simulink model "nms_3Dmodel_forward"  (R2017b)
settings: Solver=VariableStepAuto  StartTime=0.0  StopTime=t_end  FixedStep=1e-4  MinStep=1e-9  RelTol=1e-2  AbsTol=1e-3  EnableMultiTasking=on
InitFcn:
  | runScripts;
values from neighbouring files (symbols this model uses):
  ankle_height = 0.08    [nms_MechInit.m]
  ankleIMP = param(91+length(paramIC_opt):93+length(paramIC_opt))    [runScripts.m]
  c = 0.05    [IID_nms_MechInit.m]    (also in nms_MechInit.m)
  c_jointstop = 0.3 / (pi/180)    (= 17.1887338539)    [IID_nms_MechInit.m]    (also in nms_MechInit.m)
  CPG_On = 0    [setCPGPar.m]    (also in setCPGPar_inv.m = 1)
  CtrlPar_FP = [alpha0 alpha_cd alpha_cv]    [setCtrlPar.m]
  CtrlPar_FP_R = [R_hipR0 R_hipR_cd R_hipR_cv]    [setCtrlPar.m]
  CtrlPar_LL = l_clr    [setCtrlPar.m]
  CtrlPar_Side = [beta_cd  beta_cv]    [setCtrlPar.m]
  CtrlPar_St = [StPreStim St_M1 St_M2 St_M3 St_M4 St_M5 St_M11]    [setCtrlPar.m]
  CtrlPar_St_R = [R_StPreStim R_St_M1 R_St_M3 R_St_M4]    [setCtrlPar.m]
  CtrlPar_Sw = [SwPreStim SwPhasePari SwPhaseParii SwCtrlPar_H SwCtrlPar_A      SwCtrlPar_Ki SwCtrlPar_Kii SwCtrlPar_Kiii SwCtrlPar_StP]    [setCtrlPar.m]
  CtrlPar_Sw_R = [R_SwPreStim R_Sw_M6]    [setCtrlPar.m]
  CtrlPar_theta0 = parBlCtrl(1)      *1*pi/180    [setCtrlPar.m]
  CtrlPar_Tr = [Tr_St_sup Tr_Sw]    [setCtrlPar.m]
  CtrlPar_Tr_R = [R_Tr_St_sup R_Tr_Sw]    [setCtrlPar.m]
  D12_F = 0.16    [IID_nms_MechInit.m]    (also in nms_MechInit.m)
  D12_S = L_S    (= 0.5)    [IID_nms_MechInit.m]    (also in nms_MechInit.m = 0.46)
  D12_T = L_T    (= 0.5)    [IID_nms_MechInit.m]    (also in nms_MechInit.m = 0.46)
  D12z_T = 0.1* scalorFactor    (= 0.1)    [nms_MechInit.m]
  D13_F = 0.20    (= 0.2)    [IID_nms_MechInit.m]    (also in nms_MechInit.m)
  D1G_F = 0.14    [IID_nms_MechInit.m]    (also in nms_MechInit.m)
  D1G_HAT = 0.35    [IID_nms_MechInit.m]    (also in nms_MechInit.m)
  D1G_S = 0.3    [IID_nms_MechInit.m]    (also in nms_MechInit.m = 0.28)
  D1G_T = 0.3    [IID_nms_MechInit.m]    (also in nms_MechInit.m = 0.28)
  D1Gy_F = ankle_height*D1G_F/D12_F    (= 0.07)    [nms_MechInit.m]
  d_fBall = 0.1    [nms_MechInit.m]
  d_fHeel = 0.05    [nms_MechInit.m]
  DeltaThRef = 5e-3    (= 0.005)    [IID_nms_MechInit.m]    (also in nms_MechInit.m)
  Dist_LM23_PH = 0    [setDistPar.m]
  Dist_LM34_PH = 0    [setDistPar.m]
  Dist_On = 1    [IID_setDistPar.m]    (also in setDistPar.m)
  Dist_PDur = 0.15    [IID_setDistPar.m]    (also in setDistPar.m)
  Dist_RM23_PH = 0    [setDistPar.m]
  Dist_RM34_PH = 0    [setDistPar.m]
  Dist_StartTime = 15    [IID_setDistPar.m]    (also in setDistPar.m)
  Dist_xyzHAT_front_PH = 0    [setDistPar.m]
  Dist_xyzHAT_sag_PH = 0    [IID_setDistPar.m]    (also in setDistPar.m)
  Dist_xyzLAnkle_PH = 0    [setDistPar.m]
  Dist_xyzRAnkle_PH = 0    [setDistPar.m]
  eref = 0.04    [IID_nms_MechInit.m]    (also in nms_MechInit.m)
  FmaxBFSH = 350    [nms_MechInit.m]
  FmaxGAS = 1500    [IID_nms_MechInit.m]    (also in nms_MechInit.m)
  FmaxGLU = 1500    [IID_nms_MechInit.m]    (also in nms_MechInit.m)
  FmaxHAB = 3000    [nms_MechInit.m]
  FmaxHAD = 4500    [nms_MechInit.m]
  FmaxHAM = 3000    [IID_nms_MechInit.m]    (also in nms_MechInit.m)
  FmaxHFL = 2000    [IID_nms_MechInit.m]    (also in nms_MechInit.m)
  FmaxRF = 1200    [nms_MechInit.m]
  FmaxSOL = 4000    [IID_nms_MechInit.m]    (also in nms_MechInit.m)
  FmaxTA = 800    [IID_nms_MechInit.m]    (also in nms_MechInit.m)
  FmaxVAS = 6000    [IID_nms_MechInit.m]    (also in nms_MechInit.m)
  In_F = 0.005    [IID_nms_MechInit.m]    (also in nms_MechInit.m)
  In_HAT = 3    [IID_nms_MechInit.m]    (also in nms_MechInit.m = 2.5)
  In_S = 0.05    [IID_nms_MechInit.m]    (also in nms_MechInit.m)
  In_T = 0.15    [IID_nms_MechInit.m]    (also in nms_MechInit.m)
  init_a_tgt = 70*pi/180    (= 1.2217304764)    [setInitPar.m]
  init_a_tgtR = 90*pi/180    (= 1.57079632679)    [setInitPar.m]
  Inx_F = 0.0007    [nms_MechInit.m]
  Inx_HAT = 1.0    (= 1)    [nms_MechInit.m]
  Inx_S = 0.003    [nms_MechInit.m]
  Inx_T = 0.03    [nms_MechInit.m]
  Iny_F = 0.005    [nms_MechInit.m]
  Iny_HAT = 4.0    (= 4)    [nms_MechInit.m]
  Iny_S = 0.05    [nms_MechInit.m]
  Iny_T = 0.15    [nms_MechInit.m]
  K = 5    [IID_nms_MechInit.m]    (also in nms_MechInit.m)
  k_gn = k_gn/2    (= 39240)    [nms_MechInit.m]
  k_gt = k_gt/2    (= 3924)    [nms_MechInit.m]
  k_pressure = m_HAT * 9.81 / DeltaThRef    (= 104967)    [IID_nms_MechInit.m]    (also in nms_MechInit.m)
  leg_l = [D12_T D12_S]    [nms_MechInit.m]
  LongDelay = 0.020    (= 0.02)    [IID_setCtrlPar.m]    (also in nms_MechInit.m = 0.01)
  LongLoopDelay = 0.030    (= 0.03)    [nms_MechInit.m]
  loptBFSH = 0.12    [nms_MechInit.m]
  loptGAS = 0.05    [IID_nms_MechInit.m]    (also in nms_MechInit.m)
  loptGLU = 0.11    [IID_nms_MechInit.m]    (also in nms_MechInit.m)
  loptHAB = 0.09    [nms_MechInit.m]
  loptHAD = 0.10    (= 0.1)    [nms_MechInit.m]
  loptHAM = 0.10    (= 0.1)    [IID_nms_MechInit.m]    (also in nms_MechInit.m)
  loptHFL = 0.11    [IID_nms_MechInit.m]    (also in nms_MechInit.m)
  loptRF = 0.08    [nms_MechInit.m]
  loptSOL = 0.04    [IID_nms_MechInit.m]    (also in nms_MechInit.m)
  loptTA = 0.06    [IID_nms_MechInit.m]    (also in nms_MechInit.m)
  loptVAS = 0.08    [IID_nms_MechInit.m]    (also in nms_MechInit.m)
  lslackBFSH = 0.10    (= 0.1)    [nms_MechInit.m]
  lslackGAS = 0.40    (= 0.4)    [IID_nms_MechInit.m]    (also in nms_MechInit.m)
  lslackGLU = 0.13    [IID_nms_MechInit.m]    (also in nms_MechInit.m)
  lslackHAB = 0.07    [nms_MechInit.m]
  lslackHAD = 0.18    [nms_MechInit.m]
  lslackHAM = 0.31    [IID_nms_MechInit.m]    (also in nms_MechInit.m)
  lslackHFL = 0.10    (= 0.1)    [IID_nms_MechInit.m]    (also in nms_MechInit.m)
  lslackRF = 0.35    [nms_MechInit.m]
  lslackSOL = 0.26    [IID_nms_MechInit.m]    (also in nms_MechInit.m)
  lslackTA = 0.24    [IID_nms_MechInit.m]    (also in nms_MechInit.m)
  lslackVAS = 0.23    [IID_nms_MechInit.m]    (also in nms_MechInit.m)
  m_F = 1.25    [IID_nms_MechInit.m]    (also in nms_MechInit.m)
  m_HAT = 53.5    [IID_nms_MechInit.m]    (also in nms_MechInit.m)
  m_S = 3.5    [IID_nms_MechInit.m]    (also in nms_MechInit.m)
  m_T = 8.5    [IID_nms_MechInit.m]    (also in nms_MechInit.m)
  m_Total = m_F*2+m_S*2+m_T*2+m_HAT    (= 80)    [IID_nms_MechInit.m]    (also in nms_MechInit.m)
  massBFSH = 2    [nms_MechInit.m]
  massGAS = 0.45    [IID_nms_MechInit.m]    (also in nms_MechInit.m)
  massGLU = 1.4    [IID_nms_MechInit.m]    (also in nms_MechInit.m)
  massHAB = 1.145    [nms_MechInit.m]
  massHAD = 1.91    [nms_MechInit.m]
  massHAM = 1.82    [IID_nms_MechInit.m]    (also in nms_MechInit.m)
  massHFL = 1.87    [IID_nms_MechInit.m]    (also in nms_MechInit.m)
  massRF = 1    [nms_MechInit.m]
  massSOL = 1.36    [IID_nms_MechInit.m]    (also in nms_MechInit.m)
  massTA = 0.29    [IID_nms_MechInit.m]    (also in nms_MechInit.m)
  massVAS = 2.91    [IID_nms_MechInit.m]    (also in nms_MechInit.m)
  MidDelay = 0.010    (= 0.01)    [IID_setCtrlPar.m]    (also in nms_MechInit.m = 0.005)
  mu_slide = 0.8    [IID_nms_MechInit.m]    (also in nms_MechInit.m)
  mu_stick = 0.9    [IID_nms_MechInit.m]    (also in nms_MechInit.m)
  N = 1.5    [IID_nms_MechInit.m]    (also in cmaes_parfor.m = size(x,1); nms_MechInit.m)
  phi12_LowLimit = 70*pi/180    (= 1.2217304764)    [IID_nms_MechInit.m]    (also in nms_MechInit.m)
  phi12_UpLimit = 130*pi/180    (= 2.26892802759)    [IID_nms_MechInit.m]    (also in nms_MechInit.m)
  phi23_UpLimit = 175*pi/180    (= 3.05432619099)    [IID_nms_MechInit.m]    (also in nms_MechInit.m)
  phi34_UpLimit = 230*pi/180    (= 4.01425727959)    [IID_nms_MechInit.m]    (also in nms_MechInit.m)
  phi34R_LowLimit = -15*pi/180    (= -0.261799387799)    [nms_MechInit.m]
  ... (+115 more)
undefined symbols (not defined in the file or in its folder): Control_type, Fs_prosthesis, magnitude, sgn
libraries: mblibv1 x104, simulink x54, simulink_extras x38, nmc x30, NMCCPG_Library x17, powerlib_meascontrol x5
(part 2 of 17)

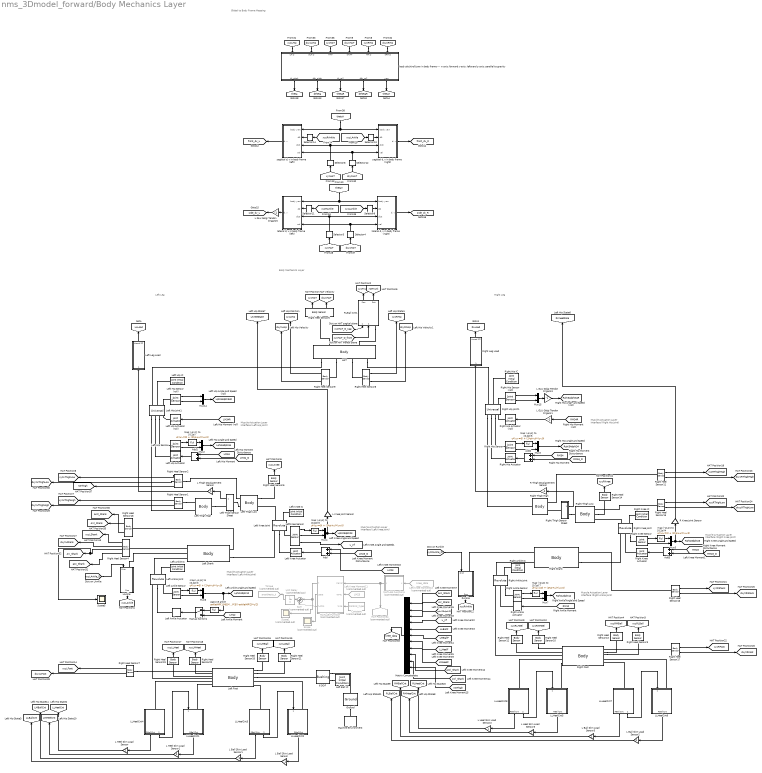
== system nms_3Dmodel_forward/Body Mechanics Layer ==
  note: Global to Body Frame Mapping
  note: Body Mechanics Layer
  note: Left Leg
  note: Right Leg
  note: Muscle Actuation
      | Layer Interface
      | (Left Hip Joint)
  note: Muscle Actuation
      | Layer Interface
      | (Left Knee Joint)
  note: Muscle Actuation
      | Layer Interface
      | (Left Ankle Joint)
  note: Muscle Actuation
      | Layer Interface
      | (Right Ankle Joint)
  note: Muscle Actuation
      | Layer Interface
      | (Right Knee Joint)
  note: Muscle Actuation
      | Layer Interface
      | (Right Hip Joint)
  6 DOF : mblibv1/Joints/Bushing  LConnTagsString=__newl0|SA1  RConnTagsString=__newr0  UpdateFromCAD=off  NumSAPorts=1  CutJoint=off  MarkAsCut=off  Primitives=prismatic_prismatic_prismatic  PrimitiveProps=P1$World$[1 0 0]$prismatic#P2$World$[0 1 0]$prismatic#P3$World$[0 0 1]$prismatic#R1$World$[1 0 0]$revolute#R2$World$[0 1 0]$revolute#R3$World$[0 0 1]$revolute  DialogClass=JointBlock  P1Axis=[1 0 0]  P2Axis=[0 1 0]  P3Axis=[0 0 1]  R1Axis=[1 0 0]  R2Axis=[0 1 0]  R3Axis=[0 0 1]
      settings: SourceProductName=Simscape Multibody  SourceProductBaseCode=MS
  Add{,1..3} (4 alike) : Sum
  Constant : Constant  Commented=on  Value=Control_type
  Ground : mblibv1/Bodies/Ground  UpdateFromCAD=off  LeftPortType=env  RightPortType=workingframe  PhysicalDomain=Mechanical  DialogClass=GroundBlock  CoordPosition=[0 0 0]  CoordPositionUnits=m  StateVectorMgrId=-1  MachineId=[0 0]  ShowEnvPort=on  ParameterChecksum=[4161457147, 3465215922, 4275957607, 1609472700]  TopologyChecksum=[2240496932, 2843436453, 1555863817, 2055023969]
      settings: SourceProductName=Simscape Multibody  SourceProductBaseCode=MS
  HAT : mblibv1/Bodies/Body  LConnTagsString=CG|CS6  RConnTagsString=CS1|CS2|CS3|CS4  UpdateFromCAD=off  DialogClass=MechanicalBodyBlock  Mass=m_HAT  MassUnits=kg  InertiaUnits=kg*m^2  Inertia=[Inx_HAT 0 0; 0 Iny_HAT 0; 0 0 In_HAT]  Shape=Cylinder  ShapeDims=[1 1]  ShapeUnits=m  ShapeUse=false  Density=1  DensityUnits=kg/m^3  DensityUse=false  GraphicsMode=MACHINE_DEFAULT  BodyColorSelMode=MACHINE_DEFAULT  BodyColor=[1 0 0]  AttachedToCS=CG  CG=Left$CG$[D1G_HAT 0 D12z_T]$CS1$CS1$m$[0 0 0]$Euler X-Y-Z$deg$WORLD$true$none  WorkingFrames=Left$CS5$[0.8 0 D12z_T]$CS1$CS1$m$[0 0 0]$Euler X-Y-Z$deg$WORLD$false$none#Right$CS1$[0 0 0]$ADJOINING$ADJOINING$m$[0 0 0]$Euler X-Y-Z$deg$WORLD$true$none#Right$CS2$[0 0 0]$CS1$CS1$m$[0 0 0]$Euler X-Y-Z$deg$WORLD$true$none#Right$CS3$[0 0 0]$CS4$CS4$m$[0 0 0]$Euler X-Y-Z$deg$WORLD$true$none#Right$CS4$[0 0 2*D12z_T]$CS1$CS1$m$[0 0 0]$Euler X-Y-Z$deg$WORLD$true$none#Left$CS6$[0 0 D12z_T]$CS1$CS1$m$[0 0 0]$Euler X-Y-Z$deg$WORLD$true$none  CGPos=[D1G_HAT 0 D12z_T]  CGRot=[0 0 0]  CS0Pos=[]  CS0Rot=[]  CS1Pos=[0 0 0]  CS1Rot=[0 0 0]  CS2Pos=[0 0 0]  CS2Rot=[0 0 0]  CS3Pos=[0 0 0]  CS3Rot=[0 0 0]  CS4Pos=[0 0 2*D12z_T]  CS4Rot=[0 0 0]  CS5Pos=[0.8 0 D12z_T]  CS5Rot=[0 0 0]  CS6Pos=[0 0 D12z_T]  CS6Rot=[0 0 0]  CS7Pos=[]  CS7Rot=[]  CS8Pos=[]  CS8Rot=[]  CS9Pos=[]  CS9Rot=[]  CS10Pos=[]  CS10Rot=[]  CS11Pos=[]  CS11Rot=[]  CS12Pos=[]  CS12Rot=[]  CS13Pos=[]  CS13Rot=[]  CS14Pos=[]  CS14Rot=[]  CS15Pos=[]  CS15Rot=[]  CS16Pos=[]  CS16Rot=[]  CS17Pos=[]  CS17Rot=[]  CS18Pos=[]  CS18Rot=[]  CS19Pos=[]  CS19Rot=[]  CS20Pos=[]  CS20Rot=[]
      settings: SourceProductName=Simscape Multibody  SourceProductBaseCode=MS
  HAT Position34 : Goto  Commented=on  GotoTag=knee_data_buffer  TagVisibility=global
  L Ball Skin Load Sensor{,1..3} (4 alike) : Gain
  L GLU Golgi Tendon Organs1 : Gain  Gain=-1
  L GLU Golgi Tendon Organs3 : Gain  Gain=-1
  L GLU Golgi Tendon Organs5 : Gain  Gain=-1
  L Heel Skin Load Sensor{,1..3} (4 alike) : Gain
  L Knee Joint Sensor : Gain
  L Thigh Displacement  Sensor : Gain
  LAnkle : Subsystem
  LLHeelCnt1 : Subsystem
  LLHeelCnt2 : Subsystem
  LLHeelCnt3 : Subsystem
  LLHeelCnt4 : Subsystem
  LLHeelCnt5 : Subsystem
  LLHeelCnt6 : Subsystem
  LLHeelCnt7 : Subsystem
  LLHeelCnt8 : Subsystem
  Left Ankle Joint : mblibv1/Joints/Revolute  LConnTagsString=__newl0|SA1|SA2  RConnTagsString=__newr0|SA1  UpdateFromCAD=off  NumSAPorts=3  CutJoint=off  MarkAsCut=off  Primitives=revolute  PrimitiveProps=R1$WORLD$[0 0 1]$revolute  DialogClass=JointBlock  R1Axis=[0 0 1]
      settings: SourceProductName=Simscape Multibody  SourceProductBaseCode=MS
  Left Hip Joint1 : mblibv1/Joints/Universal  LConnTagsString=__newl0|SA1|SA2|SA3  RConnTagsString=__newr0|SA1|SA2  UpdateFromCAD=off  NumSAPorts=5  CutJoint=off  MarkAsCut=off  Primitives=prismatic  PrimitiveProps=R1$World$[0 0 1]$revolute#R2$World$[0 1 0]$revolute  DialogClass=JointBlock  R1Axis=[0 0 1]  R2Axis=[0 1 0]
      settings: SourceProductName=Simscape Multibody  SourceProductBaseCode=MS
  Left Knee Joint : mblibv1/Joints/Revolute  LConnTagsString=__newl0|SA1|SA2  RConnTagsString=__newr0|SA1  UpdateFromCAD=off  NumSAPorts=3  CutJoint=off  MarkAsCut=off  Primitives=revolute  PrimitiveProps=R1$WORLD$[0 0 -1]$revolute  DialogClass=JointBlock  R1Axis=[0 0 -1]
      settings: SourceProductName=Simscape Multibody  SourceProductBaseCode=MS
  Left Ankle Actuator : mblibv1/Sensors &  Actuators/Joint Actuator  UpdateFromCAD=off  PhysicalDomain=Mechanical  PortType=blob  ActuationStyle=Force  AngleUnits=deg  ArcVelocityUnits=deg/s  ArcAccelerationUnits=deg/s^2  CoordPositionUnits=m  VelocityUnits=m/s  AccelerationUnits=m/s^2  ForceUnits=N  TorqueUnits=N-m  ActiveIO=on  Width=1  DialogClass=MechanicalActuatorBlock  Primitive=R1  ReferenceFrame=Absolute (INERTIAL)
      settings: SourceProductName=Simscape Multibody  SourceProductBaseCode=MS
  Left Ankle Sensor : mblibv1/Sensors &  Actuators/Joint Sensor  UpdateFromCAD=off  PhysicalDomain=Mechanical  PortType=blob  Muxed=off  Pose=off  Angle=on  AngleUnits=rad  ArcVelocity=on  ArcVelocityUnits=rad/s  ArcAcceleration=off  ArcAccelerationUnits=deg/s^2  CoordPosition=on  CoordPositionUnits=m  Velocity=off  VelocityUnits=m/s  Acceleration=off  AccelerationUnits=m/s^2  Quaternion=on  QuaternionDT=off  QuaternionDDT=off  QuaternionUnits=off  OutputVector=[ 1 1 ]  ActiveIO=on  Width=2  DialogClass=MechanicalSensorBlock  Primitive=R1  Force=off  ForceUnits=N  Torque=off  TorqueUnits=N-m  ReferenceFrame=Absolute (INERTIAL)  ReactionSensedSide=Base  ReactionReferenceFrame=Absolute (World)  ReactionForce=off  ReactionForceUnits=N  ReactionMoment=off  ReactionMomentUnits=N-m
      settings: SourceProductName=Simscape Multibody  SourceProductBaseCode=MS
  Left Ankle IC : mblibv1/Sensors &  Actuators/Joint Initial Condition  UpdateFromCAD=off  LeftPortType=blob  RightPortType=blob  PhysicalDomain=mechanical  DialogClass=InitialConditionBlock  InitialConditions=P1$false$0$m$rad$0$m/s$rad/s#P2$false$0$m$rad$0$m/s$rad/s#P3$false$0$m$rad$0$m/s$rad/s#R1$true$Lphi120$m$rad$0$m/s$rad/s#R2$false$0$m$rad$0$m/s$rad/s#R3$false$0$m$rad$0$m/s$rad/s#S$false$0$m$rad$0$m/s$rad/s  P1PIC=0  P1VIC=0  P2PIC=0  P2VIC=0  P3PIC=0  P3VIC=0  R1PIC=Lphi120  R1VIC=0  R2PIC=0  R2VIC=0  R3PIC=0  R3VIC=0  SPIC=0  SVIC=0
      settings: SourceProductName=Simscape Multibody  SourceProductBaseCode=MS
  Left Ball IC : mblibv1/Sensors &  Actuators/Joint Initial Condition  UpdateFromCAD=off  LeftPortType=blob  RightPortType=blob  PhysicalDomain=mechanical  DialogClass=InitialConditionBlock  InitialConditions=P1$true$x0$m$deg$vx0$m/s$deg/s#P2$true$z0$m$deg$0$m/s$deg/s#P3$true$-y0$m$deg$-vy0$m/s$deg/s#R1$true$roll0$m$rad$0$m/s$rad/s#R2$true$yaw0$m$rad$0$m/s$rad/s#R3$false$0$m$rad$0$m/s$rad/s#S$false$0$m$deg$0$m/s$deg/s  P1PIC=x0  P1VIC=vx0  P2PIC=z0  P2VIC=0  P3PIC=-y0  P3VIC=-vy0  R1PIC=roll0  R1VIC=0  R2PIC=yaw0  R2VIC=0  R3PIC=0  R3VIC=0  SPIC=0  SVIC=0
      settings: SourceProductName=Simscape Multibody  SourceProductBaseCode=MS
  Left Foot : mblibv1/Bodies/Body  LConnTagsString=CS3|CS4|CS1|CS5|CS6  RConnTagsString=CG|CS7|CS8|CS2|CS9|CS10  UpdateFromCAD=off  DialogClass=MechanicalBodyBlock  Mass=m_F  MassUnits=kg  InertiaUnits=kg*m^2  Inertia=[Inx_F 0 0; 0 Iny_F 0; 0 0 In_F]  Shape=Cylinder  ShapeDims=[1 1]  ShapeUnits=m  ShapeUse=false  Density=1  DensityUnits=kg/m^3  DensityUse=false  GraphicsMode=MACHINE_DEFAULT  BodyColorSelMode=MACHINE_DEFAULT  BodyColor=[1 0 0]  AttachedToCS=CG  CG=Right$CG$[-D1G_F D1Gy_F 0]$CS1$CS1$m$[0 0 0]$Euler X-Y-Z$deg$WORLD$true$none  WorkingFrames=Left$CS3$[0 0 d_fBall/2]$CS1$CS1$m$[0 0 0]$Euler X-Y-Z$deg$WORLD$true$none#Left$CS4$[0 0 -d_fBall/2]$CS1$CS1$m$[0 0 0]$Euler X-Y-Z$deg$WORLD$true$none#Right$CS7$[-D13_F 0 d_fHeel/2]$CS1$CS1$m$[0 0 0]$Euler X-Y-Z$deg$WORLD$true$none#Right$CS8$[-D13_F 0 -d_fHeel/2]$CS1$CS1$m$[0 0 0]$Euler X-Y-Z$deg$WORLD$true$none#Left$CS1$[0 0 0]$ADJOINING$ADJOINING$m$[0 0 0]$Euler X-Y-Z$deg$WORLD$true$none#Right$CS2$[-D12_F ankle_height 0]$CS1$CS1$m$[0 0 0]$Euler X-Y-Z$deg$WORLD$true$none#Left$CS5$[0 0 0]$CS4$CS4$m$[0 0 0]$Euler X-Y-Z$deg$WORLD$true$none#Left$CS6$[0 0 0]$CS3$CS3$m$[0 0 0]$Euler X-Y-Z$deg$WORLD$true$none#Right$CS9$[0 0 0]$CS8$CS8$m$[0 0 0]$Euler X-Y-Z$deg$WORLD$true$none#Right$CS10$[0 0 0]$CS7$CS7$m$[0 0 0]$Euler X-Y-Z$deg$WORLD$true$none  CGPos=[-D1G_F D1Gy_F 0]  CGRot=[0 0 0]  CS0Pos=[]  CS0Rot=[]  CS1Pos=[0 0 0]  CS1Rot=[0 0 0]  CS2Pos=[-D12_F ankle_height 0]  CS2Rot=[0 0 0]  CS3Pos=[0 0 d_fBall/2]  CS3Rot=[0 0 0]  CS4Pos=[0 0 -d_fBall/2]  CS4Rot=[0 0 0]  CS5Pos=[0 0 0]  CS5Rot=[0 0 0]  CS6Pos=[0 0 0]  CS6Rot=[0 0 0]  CS7Pos=[-D13_F 0 d_fHeel/2]  CS7Rot=[0 0 0]  CS8Pos=[-D13_F 0 -d_fHeel/2]  CS8Rot=[0 0 0]  CS9Pos=[0 0 0]  CS9Rot=[0 0 0]  CS10Pos=[0 0 0]  CS10Rot=[0 0 0]  CS11Pos=[]  CS11Rot=[]  CS12Pos=[]  CS12Rot=[]  CS13Pos=[]  CS13Rot=[]  CS14Pos=[]  CS14Rot=[]  CS15Pos=[]  CS15Rot=[]  CS16Pos=[]  CS16Rot=[]  CS17Pos=[]  CS17Rot=[]  CS18Pos=[]  CS18Rot=[]  CS19Pos=[]  CS19Rot=[]  CS20Pos=[]  CS20Rot=[]
      settings: SourceProductName=Simscape Multibody  SourceProductBaseCode=MS
  Left Hip Actuator : mblibv1/Sensors &  Actuators/Joint Actuator  UpdateFromCAD=off  PhysicalDomain=Mechanical  PortType=blob  ActuationStyle=Force  AngleUnits=deg  ArcVelocityUnits=deg/s  ArcAccelerationUnits=deg/s^2  CoordPositionUnits=m  VelocityUnits=m/s  AccelerationUnits=m/s^2  ForceUnits=N  TorqueUnits=N-m  ActiveIO=on  Width=1  DialogClass=MechanicalActuatorBlock  Primitive=R1  ReferenceFrame=Absolute (INERTIAL)
      settings: SourceProductName=Simscape Multibody  SourceProductBaseCode=MS
  Left Hip Actuator (roll) : mblibv1/Sensors &  Actuators/Joint Actuator  UpdateFromCAD=off  PhysicalDomain=Mechanical  PortType=blob  ActuationStyle=Force  AngleUnits=rad  ArcVelocityUnits=rad/s  ArcAccelerationUnits=rad/s^2  CoordPositionUnits=m  VelocityUnits=m/s  AccelerationUnits=m/s^2  ForceUnits=N  TorqueUnits=N*m  ActiveIO=on  Width=1  DialogClass=MechanicalActuatorBlock  Primitive=R2  ReferenceFrame=Absolute (INERTIAL)
      settings: SourceProductName=Simscape Multibody  SourceProductBaseCode=MS
  Left Hip Sensor : mblibv1/Sensors &  Actuators/Joint Sensor  UpdateFromCAD=off  PhysicalDomain=Mechanical  PortType=blob  Muxed=off  Pose=off  Angle=on  AngleUnits=rad  ArcVelocity=on  ArcVelocityUnits=rad/s  ArcAcceleration=off  ArcAccelerationUnits=deg/s^2  CoordPosition=on  CoordPositionUnits=m  Velocity=on  VelocityUnits=m/s  Acceleration=off  AccelerationUnits=m/s^2  Quaternion=on  QuaternionDT=off  QuaternionDDT=off  QuaternionUnits=off  OutputVector=[ 1 1 ]  ActiveIO=on  Width=2  DialogClass=MechanicalSensorBlock  Primitive=R1  Force=off  ForceUnits=N  Torque=off  TorqueUnits=N-m  ReferenceFrame=Absolute (INERTIAL)  ReactionSensedSide=Base  ReactionReferenceFrame=Absolute (World)  ReactionForce=off  ReactionForceUnits=N  ReactionMoment=off  ReactionMomentUnits=N-m
      settings: SourceProductName=Simscape Multibody  SourceProductBaseCode=MS
  Left Hip Sensor (roll) : mblibv1/Sensors &  Actuators/Joint Sensor  UpdateFromCAD=off  PhysicalDomain=Mechanical  PortType=blob  Muxed=off  Pose=off  Angle=on  AngleUnits=rad  ArcVelocity=on  ArcVelocityUnits=rad/s  ArcAcceleration=off  ArcAccelerationUnits=deg/s^2  CoordPosition=on  CoordPositionUnits=m  Velocity=on  VelocityUnits=m/s  Acceleration=off  AccelerationUnits=m/s^2  Quaternion=on  QuaternionDT=off  QuaternionDDT=off  QuaternionUnits=off  OutputVector=[ 1 1 ]  ActiveIO=on  Width=2  DialogClass=MechanicalSensorBlock  Primitive=R2  Force=off  ForceUnits=N  Torque=off  TorqueUnits=N*m  ReferenceFrame=Absolute (INERTIAL)  ReactionSensedSide=Base  ReactionReferenceFrame=Absolute (World)  ReactionForce=off  ReactionForceUnits=N  ReactionMoment=off  ReactionMomentUnits=N*m
      settings: SourceProductName=Simscape Multibody  SourceProductBaseCode=MS
  Left Hip IC : mblibv1/Sensors &  Actuators/Joint Initial Condition  UpdateFromCAD=off  LeftPortType=blob  RightPortType=blob  PhysicalDomain=mechanical  DialogClass=InitialConditionBlock  InitialConditions=P1$false$0$m$rad$0$m/s$rad/s#P2$false$0$m$rad$0$m/s$rad/s#P3$false$0$m$rad$0$m/s$rad/s#R1$true$Lphi340$m$rad$0$m/s$rad/s#R2$true$Lphi340R$m$rad$0$m/s$rad/s#R3$false$0$m$rad$0$m/s$rad/s#S$false$0$m$rad$0$m/s$rad/s  P1PIC=0  P1VIC=0  P2PIC=0  P2VIC=0  P3PIC=0  P3VIC=0  R1PIC=Lphi340  R1VIC=0  R2PIC=Lphi340R  R2VIC=0  R3PIC=0  R3VIC=0  SPIC=0  SVIC=0
      settings: SourceProductName=Simscape Multibody  SourceProductBaseCode=MS
  Left Knee Actuator : mblibv1/Sensors &  Actuators/Joint Actuator  UpdateFromCAD=off  PhysicalDomain=Mechanical  PortType=blob  ActuationStyle=Force  AngleUnits=deg  ArcVelocityUnits=deg/s  ArcAccelerationUnits=deg/s^2  CoordPositionUnits=m  VelocityUnits=m/s  AccelerationUnits=m/s^2  ForceUnits=N  TorqueUnits=N-m  ActiveIO=on  Width=1  DialogClass=MechanicalActuatorBlock  Primitive=R1  ReferenceFrame=Absolute (INERTIAL)
      settings: SourceProductName=Simscape Multibody  SourceProductBaseCode=MS
  Left Knee Moment11 : From  Commented=on  GotoTag=LM23  TagVisibility=global
      settings: CloseFcn=tagdialog Close
  Left Knee Moment13 : From  Commented=on  GotoTag=knee_data  TagVisibility=global
      settings: CloseFcn=tagdialog Close
  Left Knee IC : mblibv1/Sensors &  Actuators/Joint Initial Condition  UpdateFromCAD=off  LeftPortType=blob  RightPortType=blob  PhysicalDomain=mechanical  DialogClass=InitialConditionBlock  InitialConditions=P1$false$0$m$rad$0$m/s$rad/s#P2$false$0$m$rad$0$m/s$rad/s#P3$false$0$m$rad$0$m/s$rad/s#R1$true$Lphi230$m$rad$0$m/s$deg/s#R2$false$0$m$rad$0$m/s$rad/s#R3$false$0$m$rad$0$m/s$rad/s#S$false$0$m$rad$0$m/s$rad/s  P1PIC=0  P1VIC=0  P2PIC=0  P2VIC=0  P3PIC=0  P3VIC=0  R1PIC=Lphi230  R1VIC=0  R2PIC=0  R2VIC=0  R3PIC=0  R3VIC=0  SPIC=0  SVIC=0
      settings: SourceProductName=Simscape Multibody  SourceProductBaseCode=MS
  Left Leg Load : Subsystem
  Left Shank : mblibv1/Bodies/Body  LConnTagsString=CG|CS3|CS1  RConnTagsString=CS4|CS2  UpdateFromCAD=off  DialogClass=MechanicalBodyBlock  Mass=m_S  MassUnits=kg  InertiaUnits=kg*m^2  Inertia=[Inx_S 0 0; 0 Iny_S 0; 0 0 In_S]  Shape=Cylinder  ShapeDims=[1 1]  ShapeUnits=m  ShapeUse=false  Density=1  DensityUnits=kg/m^3  DensityUse=false  GraphicsMode=MACHINE_DEFAULT  BodyColorSelMode=MACHINE_DEFAULT  BodyColor=[1 0 0]  AttachedToCS=CG  CG=Left$CG$[D1G_S 0 0]$CS1$CS1$m$[0 0 0]$Euler X-Y-Z$deg$WORLD$true$none  WorkingFrames=Right$CS4$[D1G_S 0 0]$CS1$CS1$m$[0 0 0]$Euler X-Y-Z$deg$WORLD$true$none#Left$CS3$[0 0 0]$CS1$CS1$m$[0 0 0]$Euler X-Y-Z$deg$WORLD$true$none#Left$CS1$[0 0 0]$ADJOINING$ADJOINING$m$[0 0 0]$Euler X-Y-Z$deg$WORLD$true$none#Right$CS2$[D12_S 0 0]$CS1$CS1$m$[0 0 0]$Euler X-Y-Z$deg$WORLD$true$none  CGPos=[D1G_S 0 0]  CGRot=[0 0 0]  CS0Pos=[]  CS0Rot=[]  CS1Pos=[0 0 0]  CS1Rot=[0 0 0]  CS2Pos=[D12_S 0 0]  CS2Rot=[0 0 0]  CS3Pos=[0 0 0]  CS3Rot=[0 0 0]  CS4Pos=[D1G_S 0 0]  CS4Rot=[0 0 0]  CS5Pos=[]  CS5Rot=[]  CS6Pos=[]  CS6Rot=[]  CS7Pos=[]  CS7Rot=[]  CS8Pos=[]  CS8Rot=[]  CS9Pos=[]  CS9Rot=[]  CS10Pos=[]  CS10Rot=[]  CS11Pos=[]  CS11Rot=[]  CS12Pos=[]  CS12Rot=[]  CS13Pos=[]  CS13Rot=[]  CS14Pos=[]  CS14Rot=[]  CS15Pos=[]  CS15Rot=[]  CS16Pos=[]  CS16Rot=[]  CS17Pos=[]  CS17Rot=[]  CS18Pos=[]  CS18Rot=[]  CS19Pos=[]  CS19Rot=[]  CS20Pos=[]  CS20Rot=[]
      settings: SourceProductName=Simscape Multibody  SourceProductBaseCode=MS
  Left Thigh Sensor Sheet : Subsystem
  Left Thigh High : mblibv1/Bodies/Body  LConnTagsString=CG|CS2  RConnTagsString=CS1  UpdateFromCAD=off  DialogClass=MechanicalBodyBlock  Mass=m_T*(1-ThPos)  MassUnits=kg  InertiaUnits=kg*m^2  Inertia=[Inx_T*(1-ThPos) 0 0; 0 Iny_T*(1-ThPos)^3 0; 0 0 In_T*(1-ThPos)^3]  Shape=Cylinder  ShapeDims=[1 1]  ShapeUnits=m  ShapeUse=false  Density=1  DensityUnits=kg/m^3  DensityUse=false  GraphicsMode=MACHINE_DEFAULT  BodyColorSelMode=MACHINE_DEFAULT  BodyColor=[1 0 0]  AttachedToCS=CG  CG=Left$CG$[-D1G_T*(1-ThPos) 0 0]$CS1$CS1$m$[0 0 0]$Euler X-Y-Z$deg$WORLD$true$none  WorkingFrames=Right$CS1$[0 0 0]$ADJOINING$ADJOINING$m$[0 0 0]$Euler X-Y-Z$deg$WORLD$true$none#Left$CS2$[-D12_T*(1-ThPos) 0 0]$CS1$CS1$m$[0 0 0]$Euler X-Y-Z$deg$WORLD$true$none  CGPos=[-D1G_T*(1-ThPos) 0 0]  CGRot=[0 0 0]  CS0Pos=[]  CS0Rot=[]  CS1Pos=[0 0 0]  CS1Rot=[0 0 0]  CS2Pos=[-D12_T*(1-ThPos) 0 0]  CS2Rot=[0 0 0]  CS3Pos=[]  CS3Rot=[]  CS4Pos=[]  CS4Rot=[]  CS5Pos=[]  CS5Rot=[]  CS6Pos=[]  CS6Rot=[]  CS7Pos=[]  CS7Rot=[]  CS8Pos=[]  CS8Rot=[]  CS9Pos=[]  CS9Rot=[]  CS10Pos=[]  CS10Rot=[]  CS11Pos=[]  CS11Rot=[]  CS12Pos=[]  CS12Rot=[]  CS13Pos=[]  CS13Rot=[]  CS14Pos=[]  CS14Rot=[]  CS15Pos=[]  CS15Rot=[]  CS16Pos=[]  CS16Rot=[]  CS17Pos=[]  CS17Rot=[]  CS18Pos=[]  CS18Rot=[]  CS19Pos=[]  CS19Rot=[]  CS20Pos=[]  CS20Rot=[]
      settings: SourceProductName=Simscape Multibody  SourceProductBaseCode=MS
  Left Thigh Low : mblibv1/Bodies/Body  LConnTagsString=CG|CS2  RConnTagsString=CS3|CS1  UpdateFromCAD=off  DialogClass=MechanicalBodyBlock  Mass=m_T*ThPos  MassUnits=kg  InertiaUnits=kg*m^2  Inertia=[Inx_T*ThPos 0 0; 0 Iny_T*(ThPos)^3 0; 0 0 In_T*(ThPos)^3]  Shape=Cylinder  ShapeDims=[1 1]  ShapeUnits=m  ShapeUse=false  Density=1  DensityUnits=kg/m^3  DensityUse=false  GraphicsMode=MACHINE_DEFAULT  BodyColorSelMode=MACHINE_DEFAULT  BodyColor=[1 0 0]  AttachedToCS=CG  CG=Left$CG$[-D1G_T*ThPos 0 0]$CS1$CS1$m$[0 0 0]$Euler X-Y-Z$deg$WORLD$true$none  WorkingFrames=Right$CS3$[0 0 0]$CS1$CS1$m$[0 0 0]$Euler X-Y-Z$deg$WORLD$true$none#Right$CS1$[0 0 0]$ADJOINING$ADJOINING$m$[0 0 0]$Euler X-Y-Z$deg$WORLD$true$none#Left$CS2$[-D12_T*ThPos 0 0]$CS1$CS1$m$[0 0 0]$Euler X-Y-Z$deg$WORLD$true$none  CGPos=[-D1G_T*ThPos 0 0]  CGRot=[0 0 0]  CS0Pos=[]  CS0Rot=[]  CS1Pos=[0 0 0]  CS1Rot=[0 0 0]  CS2Pos=[-D12_T*ThPos 0 0]  CS2Rot=[0 0 0]  CS3Pos=[0 0 0]  CS3Rot=[0 0 0]  CS4Pos=[]  CS4Rot=[]  CS5Pos=[]  CS5Rot=[]  CS6Pos=[]  CS6Rot=[]  CS7Pos=[]  CS7Rot=[]  CS8Pos=[]  CS8Rot=[]  CS9Pos=[]  CS9Rot=[]  CS10Pos=[]  CS10Rot=[]  CS11Pos=[]  CS11Rot=[]  CS12Pos=[]  CS12Rot=[]  CS13Pos=[]  CS13Rot=[]  CS14Pos=[]  CS14Rot=[]  CS15Pos=[]  CS15Rot=[]  CS16Pos=[]  CS16Rot=[]  CS17Pos=[]  CS17Rot=[]  CS18Pos=[]  CS18Rot=[]  CS19Pos=[]  CS19Rot=[]  CS20Pos=[]  CS20Rot=[]
      settings: SourceProductName=Simscape Multibody  SourceProductBaseCode=MS
  LeftKnee Sensor : mblibv1/Sensors &  Actuators/Joint Sensor  UpdateFromCAD=off  PhysicalDomain=Mechanical  PortType=blob  Muxed=off  Pose=off  Angle=on  AngleUnits=rad  ArcVelocity=on  ArcVelocityUnits=rad/s  ArcAcceleration=off  ArcAccelerationUnits=deg/s^2  CoordPosition=on  CoordPositionUnits=m  Velocity=off  VelocityUnits=m/s  Acceleration=off  AccelerationUnits=m/s^2  Quaternion=on  QuaternionDT=off  QuaternionDDT=off  QuaternionUnits=off  OutputVector=[ 1 1 ]  ActiveIO=on  Width=5  DialogClass=MechanicalSensorBlock  Primitive=R1  Force=off  ForceUnits=N  Torque=off  TorqueUnits=N*m  ReferenceFrame=Absolute (INERTIAL)  ReactionSensedSide=Base  ReactionReferenceFrame=Absolute (World)  ReactionForce=on  ReactionForceUnits=N  ReactionMoment=off  ReactionMomentUnits=N*m
      settings: SourceProductName=Simscape Multibody  SourceProductBaseCode=MS
  MATLAB Function : MATLAB Function  Commented=on  TreatAsAtomicUnit=on
  MATLAB Function1 : MATLAB Function  Commented=on  TreatAsAtomicUnit=on
  Machine Environment : mblibv1/Bodies/Machine Environment  Tag=Factory ground  PortType=env  PhysicalDomain=Mechanical  DialogTemplateClass=MECH.MachineEnvironment  SyncWhenCopied=off  Gravity=[0 -9.81 0]  GravityUnits=m/s^2  GravityAsSignal=off  Dimensionality=3D Only  AnalysisType=Forward dynamics  LinearAssemblyTolerance=1e-3  LinearAssemblyToleranceUnits=m  AngularAssemblyTolerance=1e-3  AngularAssemblyToleranceUnits=rad  ConstraintSolverType=Tolerancing  ConstraintRelTolerance=1e-3  ConstraintAbsTolerance=1e-3  UseRobustSingularityHandling=off  RedundancyAnalysisToleranceType=Automatically select tolerance  RedundancyAnalysisTolerance=1e-14  StatePerturbationType=Fixed  PerturbationSize=1e-3  VisualizeMachine=on  BodyVisualizationType=Use model default body geometries  BodyColorSelMode=Use model default  DefaultBodyColor=[1 0.65 0]
      settings: SourceProductName=Simscape Multibody  SourceProductBaseCode=MS
  Manual Switch1 : ManualSwitch
  Matrix Concatenate : Concatenate  NumInputs=11  ConcatenateDimension=2
  Mux{2..7,14..15} (8 alike) : Mux  Inputs=2
  R Knee Joint Sensor : Gain
  R Thigh Displacement  Sensor : Gain  Gain=-1
  RAnkle : Subsystem
  RLBall Cnt1 : Subsystem
  Right Ankle Joint : mblibv1/Joints/Revolute  LConnTagsString=__newl0|SA1|SA2  RConnTagsString=__newr0|SA1  UpdateFromCAD=off  NumSAPorts=3  CutJoint=off  MarkAsCut=off  Primitives=revolute  PrimitiveProps=R1$WORLD$[0 0 1]$revolute  DialogClass=JointBlock  R1Axis=[0 0 1]
      settings: SourceProductName=Simscape Multibody  SourceProductBaseCode=MS
  Right Hip Joint1 : mblibv1/Joints/Universal  LConnTagsString=__newl0|SA1|SA2|SA3  RConnTagsString=__newr0|SA1|SA2  UpdateFromCAD=off  NumSAPorts=5  CutJoint=off  MarkAsCut=off  Primitives=prismatic  PrimitiveProps=R1$World$[0 0 1]$revolute#R2$World$[0 1 0]$revolute  DialogClass=JointBlock  R1Axis=[0 0 1]  R2Axis=[0 1 0]
      settings: SourceProductName=Simscape Multibody  SourceProductBaseCode=MS
  Right Knee Joint : mblibv1/Joints/Revolute  LConnTagsString=__newl0|SA1|SA2  RConnTagsString=__newr0|SA1  UpdateFromCAD=off  NumSAPorts=3  CutJoint=off  MarkAsCut=off  Primitives=revolute  PrimitiveProps=R1$WORLD$[0 0 -1]$revolute  DialogClass=JointBlock  R1Axis=[0 0 -1]
      settings: SourceProductName=Simscape Multibody  SourceProductBaseCode=MS
  Right Ankle Actuator : mblibv1/Sensors &  Actuators/Joint Actuator  UpdateFromCAD=off  PhysicalDomain=Mechanical  PortType=blob  ActuationStyle=Force  AngleUnits=deg  ArcVelocityUnits=deg/s  ArcAccelerationUnits=deg/s^2  CoordPositionUnits=m  VelocityUnits=m/s  AccelerationUnits=m/s^2  ForceUnits=N  TorqueUnits=N-m  ActiveIO=on  Width=1  DialogClass=MechanicalActuatorBlock  Primitive=R1  ReferenceFrame=Absolute (INERTIAL)
      settings: SourceProductName=Simscape Multibody  SourceProductBaseCode=MS
  Right Ankle Sensor : mblibv1/Sensors &  Actuators/Joint Sensor  UpdateFromCAD=off  PhysicalDomain=Mechanical  PortType=blob  Muxed=off  Pose=off  Angle=on  AngleUnits=rad  ArcVelocity=on  ArcVelocityUnits=rad/s  ArcAcceleration=off  ArcAccelerationUnits=deg/s^2  CoordPosition=on  CoordPositionUnits=m  Velocity=off  VelocityUnits=m/s  Acceleration=off  AccelerationUnits=m/s^2  Quaternion=on  QuaternionDT=off  QuaternionDDT=off  QuaternionUnits=off  OutputVector=[ 1 1 ]  ActiveIO=on  Width=2  DialogClass=MechanicalSensorBlock  Primitive=R1  Force=off  ForceUnits=N  Torque=off  TorqueUnits=N-m  ReferenceFrame=Absolute (INERTIAL)  ReactionSensedSide=Base  ReactionReferenceFrame=Absolute (World)  ReactionForce=off  ReactionForceUnits=N  ReactionMoment=off  ReactionMomentUnits=N-m
      settings: SourceProductName=Simscape Multibody  SourceProductBaseCode=MS
  Right Ankle IC : mblibv1/Sensors &  Actuators/Joint Initial Condition  UpdateFromCAD=off  LeftPortType=blob  RightPortType=blob  PhysicalDomain=mechanical  DialogClass=InitialConditionBlock  InitialConditions=P1$false$0$m$rad$0$m/s$rad/s#P2$false$0$m$rad$0$m/s$rad/s#P3$false$0$m$rad$0$m/s$rad/s#R1$true$Rphi120$m$rad$0$m/s$rad/s#R2$false$0$m$rad$0$m/s$rad/s#R3$false$0$m$rad$0$m/s$rad/s#S$false$0$m$rad$0$m/s$rad/s  P1PIC=0  P1VIC=0  P2PIC=0  P2VIC=0  P3PIC=0  P3VIC=0  R1PIC=Rphi120  R1VIC=0  R2PIC=0  R2VIC=0  R3PIC=0  R3VIC=0  SPIC=0  SVIC=0
      settings: SourceProductName=Simscape Multibody  SourceProductBaseCode=MS
  Right Foot : mblibv1/Bodies/Body  LConnTagsString=CG|CS3|CS4|CS2|CS5|CS6  RConnTagsString=CS7|CS8|CS1|CS9|CS10  UpdateFromCAD=off  DialogClass=MechanicalBodyBlock  Mass=m_F  MassUnits=kg  InertiaUnits=kg*m^2  Inertia=[Inx_F 0 0; 0 Iny_F 0; 0 0 In_F]  Shape=Cylinder  ShapeDims=[1 1]  ShapeUnits=m  ShapeUse=false  Density=1  DensityUnits=kg/m^3  DensityUse=false  GraphicsMode=MACHINE_DEFAULT  BodyColorSelMode=MACHINE_DEFAULT  BodyColor=[1 0 0]  AttachedToCS=CG  CG=Left$CG$[-D1G_F D1Gy_F 0]$CS2$CS2$m$[0 0 0]$Euler X-Y-Z$deg$WORLD$true$none  WorkingFrames=Left$CS3$[0 0 -d_fBall/2]$CS2$CS2$m$[0 0 0]$Euler X-Y-Z$deg$WORLD$true$none#Left$CS4$[0 0 d_fBall/2]$CS2$CS2$m$[0 0 0]$Euler X-Y-Z$deg$WORLD$true$none#Right$CS7$[-D13_F 0 -d_fHeel/2]$CS2$CS2$m$[0 0 0]$Euler X-Y-Z$deg$WORLD$true$none#Right$CS8$[-D13_F 0 d_fHeel/2]$CS2$CS2$m$[0 0 0]$Euler X-Y-Z$deg$WORLD$true$none#Right$CS1$[0 0 0]$ADJOINING$ADJOINING$m$[0 0 0]$Euler X-Y-Z$deg$WORLD$true$none#Left$CS2$[D12_F -ankle_height 0]$CS1$CS1$m$[0 0 0]$Euler X-Y-Z$deg$WORLD$true$none#Left$CS5$[0 0 0]$CS4$CS4$m$[0 0 0]$Euler X-Y-Z$deg$WORLD$true$none#Left$CS6$[0 0 0]$CS3$CS3$m$[0 0 0]$Euler X-Y-Z$deg$WORLD$true$none#Right$CS9$[0 0 0]$CS8$CS8$m$[0 0 0]$Euler X-Y-Z$deg$WORLD$true$none#Right$CS10$[0 0 0]$CS7$CS7$m$[0 0 0]$Euler X-Y-Z$deg$WORLD$true$none  CGPos=[-D1G_F D1Gy_F 0]  CGRot=[0 0 0]  CS0Pos=[]  CS0Rot=[]  CS1Pos=[0 0 0]  CS1Rot=[0 0 0]  CS2Pos=[D12_F -ankle_height 0]  CS2Rot=[0 0 0]  CS3Pos=[0 0 -d_fBall/2]  CS3Rot=[0 0 0]  CS4Pos=[0 0 d_fBall/2]  CS4Rot=[0 0 0]  CS5Pos=[0 0 0]  CS5Rot=[0 0 0]  CS6Pos=[0 0 0]  CS6Rot=[0 0 0]  CS7Pos=[-D13_F 0 -d_fHeel/2]  CS7Rot=[0 0 0]  CS8Pos=[-D13_F 0 d_fHeel/2]  CS8Rot=[0 0 0]  CS9Pos=[0 0 0]  CS9Rot=[0 0 0]  CS10Pos=[0 0 0]  CS10Rot=[0 0 0]  CS11Pos=[]  CS11Rot=[]  CS12Pos=[]  CS12Rot=[]  CS13Pos=[]  CS13Rot=[]  CS14Pos=[]  CS14Rot=[]  CS15Pos=[]  CS15Rot=[]  CS16Pos=[]  CS16Rot=[]  CS17Pos=[]  CS17Rot=[]  CS18Pos=[]  CS18Rot=[]  CS19Pos=[]  CS19Rot=[]  CS20Pos=[]  CS20Rot=[]
      settings: SourceProductName=Simscape Multibody  SourceProductBaseCode=MS
  Right Heel Sensor{1,5,7..9,11,15..17} (9 alike) : mblibv1/Sensors &  Actuators/Body Sensor  UpdateFromCAD=off  PhysicalDomain=Mechanical  PortType=blob  Muxed=off  Pose=off  Angle=on  AngleUnits=deg  ArcVelocity=off  ArcVelocityUnits=deg/s  ArcAcceleration=off  ArcAccelerationUnits=deg/s^2  CoordPosition=on  CoordPositionUnits=m  Velocity=on  VelocityUnits=m/s  Acceleration=off  AccelerationUnits=m/s^2  Quaternion=on  QuaternionDT=off  QuaternionDDT=off  QuaternionUnits=off  OutputVector=[ 3 3 ]  ActiveIO=on  Width=6  DialogClass=MechanicalSensorBlock  ReferenceFrame=Absolute (World)
      settings: SourceProductName=Simscape Multibody  SourceProductBaseCode=MS
  Right Heel Sensor{3,6,10,12..14,20..23} (10 alike) : mblibv1/Sensors &  Actuators/Body Sensor  UpdateFromCAD=off  PhysicalDomain=Mechanical  PortType=blob  Muxed=off  Pose=off  Angle=on  AngleUnits=deg  ArcVelocity=off  ArcVelocityUnits=deg/s  ArcAcceleration=off  ArcAccelerationUnits=deg/s^2  CoordPosition=on  CoordPositionUnits=m  Velocity=off  VelocityUnits=m/s  Acceleration=off  AccelerationUnits=m/s^2  Quaternion=on  QuaternionDT=off  QuaternionDDT=off  QuaternionUnits=off  OutputVector=[ 3 3 ]  ActiveIO=on  Width=3  DialogClass=MechanicalSensorBlock  ReferenceFrame=Absolute (World)
      settings: SourceProductName=Simscape Multibody  SourceProductBaseCode=MS
  Right Heel Sensor18 : mblibv1/Sensors &  Actuators/Body Sensor  UpdateFromCAD=off  PhysicalDomain=Mechanical  PortType=blob  Muxed=off  Pose=off  Angle=on  AngleUnits=deg  ArcVelocity=on  ArcVelocityUnits=deg/s  ArcAcceleration=off  ArcAccelerationUnits=deg/s^2  CoordPosition=off  CoordPositionUnits=m  Velocity=off  VelocityUnits=m/s  Acceleration=on  AccelerationUnits=m/s^2  Quaternion=on  QuaternionDT=off  QuaternionDDT=off  QuaternionUnits=off  OutputVector=[ 3 3 ]  ActiveIO=on  Width=6  DialogClass=MechanicalSensorBlock  ReferenceFrame=Local (Body CS)
      settings: SourceProductName=Simscape Multibody  SourceProductBaseCode=MS
  Right Heel Sensor2 : mblibv1/Sensors &  Actuators/Body Sensor  UpdateFromCAD=off  PhysicalDomain=Mechanical  PortType=blob  Muxed=off  Pose=on  Angle=on  AngleUnits=deg  ArcVelocity=off  ArcVelocityUnits=deg/s  ArcAcceleration=off  ArcAccelerationUnits=deg/s^2  CoordPosition=on  CoordPositionUnits=m  Velocity=on  VelocityUnits=m/s  Acceleration=off  AccelerationUnits=m/s^2  Quaternion=on  QuaternionDT=off  QuaternionDDT=off  QuaternionUnits=off  OutputVector=[ 3 3 ]  ActiveIO=on  Width=15  DialogClass=MechanicalSensorBlock  ReferenceFrame=Absolute (World)
      settings: SourceProductName=Simscape Multibody  SourceProductBaseCode=MS
  Right Heel Sensor4 : mblibv1/Sensors &  Actuators/Body Sensor  UpdateFromCAD=off  PhysicalDomain=Mechanical  PortType=blob  Muxed=off  Pose=off  Angle=on  AngleUnits=deg  ArcVelocity=on  ArcVelocityUnits=deg/s  ArcAcceleration=off  ArcAccelerationUnits=deg/s^2  CoordPosition=on  CoordPositionUnits=m  Velocity=on  VelocityUnits=m/s  Acceleration=on  AccelerationUnits=m/s^2  Quaternion=on  QuaternionDT=off  QuaternionDDT=off  QuaternionUnits=off  OutputVector=[ 3 3 ]  ActiveIO=on  Width=12  DialogClass=MechanicalSensorBlock  ReferenceFrame=Absolute (World)
      settings: SourceProductName=Simscape Multibody  SourceProductBaseCode=MS
  Right Hip Actuator : mblibv1/Sensors &  Actuators/Joint Actuator  UpdateFromCAD=off  PhysicalDomain=Mechanical  PortType=blob  ActuationStyle=Force  AngleUnits=deg  ArcVelocityUnits=deg/s  ArcAccelerationUnits=deg/s^2  CoordPositionUnits=m  VelocityUnits=m/s  AccelerationUnits=m/s^2  ForceUnits=N  TorqueUnits=N-m  ActiveIO=on  Width=1  DialogClass=MechanicalActuatorBlock  Primitive=R1  ReferenceFrame=Absolute (INERTIAL)
      settings: SourceProductName=Simscape Multibody  SourceProductBaseCode=MS
  Right Hip Actuator (roll) : mblibv1/Sensors &  Actuators/Joint Actuator  UpdateFromCAD=off  PhysicalDomain=Mechanical  PortType=blob  ActuationStyle=Force  AngleUnits=rad  ArcVelocityUnits=rad/s  ArcAccelerationUnits=rad/s^2  CoordPositionUnits=m  VelocityUnits=m/s  AccelerationUnits=m/s^2  ForceUnits=N  TorqueUnits=N*m  ActiveIO=on  Width=1  DialogClass=MechanicalActuatorBlock  Primitive=R2  ReferenceFrame=Absolute (INERTIAL)
      settings: SourceProductName=Simscape Multibody  SourceProductBaseCode=MS
  Right Hip Sensor : mblibv1/Sensors &  Actuators/Joint Sensor  UpdateFromCAD=off  PhysicalDomain=Mechanical  PortType=blob  Muxed=off  Pose=off  Angle=on  AngleUnits=rad  ArcVelocity=on  ArcVelocityUnits=rad/s  ArcAcceleration=off  ArcAccelerationUnits=deg/s^2  CoordPosition=on  CoordPositionUnits=m  Velocity=on  VelocityUnits=m/s  Acceleration=off  AccelerationUnits=m/s^2  Quaternion=on  QuaternionDT=off  QuaternionDDT=off  QuaternionUnits=off  OutputVector=[ 1 1 ]  ActiveIO=on  Width=2  DialogClass=MechanicalSensorBlock  Primitive=R1  Force=off  ForceUnits=N  Torque=off  TorqueUnits=N-m  ReferenceFrame=Absolute (INERTIAL)  ReactionSensedSide=Base  ReactionReferenceFrame=Absolute (World)  ReactionForce=off  ReactionForceUnits=N  ReactionMoment=off  ReactionMomentUnits=N-m
      settings: SourceProductName=Simscape Multibody  SourceProductBaseCode=MS
  Right Hip Sensor (roll) : mblibv1/Sensors &  Actuators/Joint Sensor  UpdateFromCAD=off  PhysicalDomain=Mechanical  PortType=blob  Muxed=off  Pose=off  Angle=on  AngleUnits=rad  ArcVelocity=on  ArcVelocityUnits=rad/s  ArcAcceleration=off  ArcAccelerationUnits=deg/s^2  CoordPosition=on  CoordPositionUnits=m  Velocity=on  VelocityUnits=m/s  Acceleration=off  AccelerationUnits=m/s^2  Quaternion=on  QuaternionDT=off  QuaternionDDT=off  QuaternionUnits=off  OutputVector=[ 1 1 ]  ActiveIO=on  Width=2  DialogClass=MechanicalSensorBlock  Primitive=R2  Force=off  ForceUnits=N  Torque=off  TorqueUnits=N*m  ReferenceFrame=Absolute (INERTIAL)  ReactionSensedSide=Base  ReactionReferenceFrame=Absolute (World)  ReactionForce=off  ReactionForceUnits=N  ReactionMoment=off  ReactionMomentUnits=N*m
      settings: SourceProductName=Simscape Multibody  SourceProductBaseCode=MS
  Right Hip IC : mblibv1/Sensors &  Actuators/Joint Initial Condition  UpdateFromCAD=off  LeftPortType=blob  RightPortType=blob  PhysicalDomain=mechanical  DialogClass=InitialConditionBlock  InitialConditions=P1$false$0$m$rad$0$m/s$rad/s#P2$false$0$m$rad$0$m/s$rad/s#P3$false$0$m$rad$0$m/s$rad/s#R1$true$Rphi340$m$rad$0$m/s$rad/s#R2$true$-Rphi340R$m$rad$0$m/s$rad/s#R3$false$0$m$rad$0$m/s$rad/s#S$false$0$m$rad$0$m/s$rad/s  P1PIC=0  P1VIC=0  P2PIC=0  P2VIC=0  P3PIC=0  P3VIC=0  R1PIC=Rphi340  R1VIC=0  R2PIC=-Rphi340R  R2VIC=0  R3PIC=0  R3VIC=0  SPIC=0  SVIC=0
      settings: SourceProductName=Simscape Multibody  SourceProductBaseCode=MS
  Right Knee Actuator : mblibv1/Sensors &  Actuators/Joint Actuator  UpdateFromCAD=off  PhysicalDomain=Mechanical  PortType=blob  ActuationStyle=Force  AngleUnits=deg  ArcVelocityUnits=deg/s  ArcAccelerationUnits=deg/s^2  CoordPositionUnits=m  VelocityUnits=m/s  AccelerationUnits=m/s^2  ForceUnits=N  TorqueUnits=N-m  ActiveIO=on  Width=1  DialogClass=MechanicalActuatorBlock  Primitive=R1  ReferenceFrame=Absolute (INERTIAL)
      settings: SourceProductName=Simscape Multibody  SourceProductBaseCode=MS
  Right Knee Sensor : mblibv1/Sensors &  Actuators/Joint Sensor  UpdateFromCAD=off  PhysicalDomain=Mechanical  PortType=blob  Muxed=off  Pose=off  Angle=on  AngleUnits=rad  ArcVelocity=on  ArcVelocityUnits=rad/s  ArcAcceleration=off  ArcAccelerationUnits=deg/s^2  CoordPosition=on  CoordPositionUnits=m  Velocity=off  VelocityUnits=m/s  Acceleration=off  AccelerationUnits=m/s^2  Quaternion=on  QuaternionDT=off  QuaternionDDT=off  QuaternionUnits=off  OutputVector=[ 1 1 ]  ActiveIO=on  Width=2  DialogClass=MechanicalSensorBlock  Primitive=R1  Force=off  ForceUnits=N  Torque=off  TorqueUnits=N-m  ReferenceFrame=Absolute (INERTIAL)  ReactionSensedSide=Base  ReactionReferenceFrame=Absolute (World)  ReactionForce=off  ReactionForceUnits=N  ReactionMoment=off  ReactionMomentUnits=N-m
      settings: SourceProductName=Simscape Multibody  SourceProductBaseCode=MS
  Right Knee IC : mblibv1/Sensors &  Actuators/Joint Initial Condition  UpdateFromCAD=off  LeftPortType=blob  RightPortType=blob  PhysicalDomain=mechanical  DialogClass=InitialConditionBlock  InitialConditions=P1$false$0$m$rad$0$m/s$rad/s#P2$false$0$m$rad$0$m/s$rad/s#P3$false$0$m$rad$0$m/s$rad/s#R1$true$Rphi230$m$rad$0$m/s$rad/s#R2$false$0$m$rad$0$m/s$rad/s#R3$false$0$m$rad$0$m/s$rad/s#S$false$0$m$rad$0$m/s$rad/s  P1PIC=0  P1VIC=0  P2PIC=0  P2VIC=0  P3PIC=0  P3VIC=0  R1PIC=Rphi230  R1VIC=0  R2PIC=0  R2VIC=0  R3PIC=0  R3VIC=0  SPIC=0  SVIC=0
      settings: SourceProductName=Simscape Multibody  SourceProductBaseCode=MS
  Right Leg Load : Subsystem
  Right Shank : mblibv1/Bodies/Body  LConnTagsString=CS3|CS2  RConnTagsString=CG|CS1  UpdateFromCAD=off  DialogClass=MechanicalBodyBlock  Mass=m_S  MassUnits=kg  InertiaUnits=kg*m^2  Inertia=[Inx_S 0 0; 0 Iny_S 0; 0 0 In_S]  Shape=Cylinder  ShapeDims=[1 1]  ShapeUnits=m  ShapeUse=false  Density=1  DensityUnits=kg/m^3  DensityUse=false  GraphicsMode=MACHINE_DEFAULT  BodyColorSelMode=MACHINE_DEFAULT  BodyColor=[1 0 0]  AttachedToCS=CG  CG=Right$CG$[D1G_S 0 0]$CS2$CS2$m$[0 0 0]$Euler X-Y-Z$deg$WORLD$true$none  WorkingFrames=Left$CS3$[0 0 0]$CS2$CS2$m$[0 0 0]$Euler X-Y-Z$deg$WORLD$true$none#Right$CS1$[0 0 0]$ADJOINING$ADJOINING$m$[0 0 0]$Euler X-Y-Z$deg$WORLD$true$none#Left$CS2$[-D12_S 0 0]$CS1$CS1$m$[0 0 0]$Euler X-Y-Z$deg$WORLD$true$none  CGPos=[D1G_S 0 0]  CGRot=[0 0 0]  CS0Pos=[]  CS0Rot=[]  CS1Pos=[0 0 0]  CS1Rot=[0 0 0]  CS2Pos=[-D12_S 0 0]  CS2Rot=[0 0 0]  CS3Pos=[0 0 0]  CS3Rot=[0 0 0]  CS4Pos=[]  CS4Rot=[]  CS5Pos=[]  CS5Rot=[]  CS6Pos=[]  CS6Rot=[]  CS7Pos=[]  CS7Rot=[]  CS8Pos=[]  CS8Rot=[]  CS9Pos=[]  CS9Rot=[]  CS10Pos=[]  CS10Rot=[]  CS11Pos=[]  CS11Rot=[]  CS12Pos=[]  CS12Rot=[]  CS13Pos=[]  CS13Rot=[]  CS14Pos=[]  CS14Rot=[]  CS15Pos=[]  CS15Rot=[]  CS16Pos=[]  CS16Rot=[]  CS17Pos=[]  CS17Rot=[]  CS18Pos=[]  CS18Rot=[]  CS19Pos=[]  CS19Rot=[]  CS20Pos=[]  CS20Rot=[]
      settings: SourceProductName=Simscape Multibody  SourceProductBaseCode=MS
  Right Thigh Sensor Sheet : Subsystem
  Right Thigh High : mblibv1/Bodies/Body  LConnTagsString=CG|CS2  RConnTagsString=CS1  UpdateFromCAD=off  DialogClass=MechanicalBodyBlock  Mass=m_T*(1-ThPos)  MassUnits=kg  InertiaUnits=kg*m^2  Inertia=[Inx_T*(1-ThPos) 0 0; 0 Iny_T*(1-ThPos)^3 0; 0 0 In_T*(1-ThPos)^3]  Shape=Cylinder  ShapeDims=[1 1]  ShapeUnits=m  ShapeUse=false  Density=1  DensityUnits=kg/m^3  DensityUse=false  GraphicsMode=MACHINE_DEFAULT  BodyColorSelMode=MACHINE_DEFAULT  BodyColor=[1 0 0]  AttachedToCS=CG  CG=Left$CG$[-D1G_T*(1-ThPos) 0 0]$CS2$CS2$m$[0 0 0]$Euler X-Y-Z$deg$WORLD$true$none  WorkingFrames=Right$CS1$[0 0 0]$Adjoining$Adjoining$m$[0 0 0]$Euler X-Y-Z$deg$WORLD$true$none#Left$CS2$[D12_T*(1-ThPos) 0 0]$CS1$CS1$m$[0 0 0]$Euler X-Y-Z$deg$WORLD$true$none  CGPos=[-D1G_T*(1-ThPos) 0 0]  CGRot=[0 0 0]  CS0Pos=[]  CS0Rot=[]  CS1Pos=[0 0 0]  CS1Rot=[0 0 0]  CS2Pos=[D12_T*(1-ThPos) 0 0]  CS2Rot=[0 0 0]  CS3Pos=[]  CS3Rot=[]  CS4Pos=[]  CS4Rot=[]  CS5Pos=[]  CS5Rot=[]  CS6Pos=[]  CS6Rot=[]  CS7Pos=[]  CS7Rot=[]  CS8Pos=[]  CS8Rot=[]  CS9Pos=[]  CS9Rot=[]  CS10Pos=[]  CS10Rot=[]  CS11Pos=[]  CS11Rot=[]  CS12Pos=[]  CS12Rot=[]  CS13Pos=[]  CS13Rot=[]  CS14Pos=[]  CS14Rot=[]  CS15Pos=[]  CS15Rot=[]  CS16Pos=[]  CS16Rot=[]  CS17Pos=[]  CS17Rot=[]  CS18Pos=[]  CS18Rot=[]  CS19Pos=[]  CS19Rot=[]  CS20Pos=[]  CS20Rot=[]
      settings: SourceProductName=Simscape Multibody  SourceProductBaseCode=MS
  Right Thigh Low : mblibv1/Bodies/Body  LConnTagsString=CG|CS3|CS2  RConnTagsString=CS1  UpdateFromCAD=off  DialogClass=MechanicalBodyBlock  Mass=m_T*ThPos  MassUnits=kg  InertiaUnits=kg*m^2  Inertia=[Inx_T*ThPos 0 0; 0 Iny_T*(ThPos)^3 0; 0 0 In_T*(ThPos)^3]  Shape=Cylinder  ShapeDims=[1 1]  ShapeUnits=m  ShapeUse=false  Density=1  DensityUnits=kg/m^3  DensityUse=false  GraphicsMode=MACHINE_DEFAULT  BodyColorSelMode=MACHINE_DEFAULT  BodyColor=[1 0 0]  AttachedToCS=CG  CG=Left$CG$[-D1G_T*ThPos 0 0]$CS2$CS2$m$[0 0 0]$Euler X-Y-Z$deg$WORLD$true$none  WorkingFrames=Right$CS1$[0 0 0]$ADJOINING$ADJOINING$m$[0 0 0]$Euler X-Y-Z$deg$WORLD$true$none#Left$CS3$[0 0 0]$CS2$CS2$m$[0 0 0]$Euler X-Y-Z$deg$WORLD$true$none#Left$CS2$[D12_T*ThPos 0 0]$CS1$CS1$m$[0 0 0]$Euler X-Y-Z$deg$WORLD$true$none  CGPos=[-D1G_T*ThPos 0 0]  CGRot=[0 0 0]  CS0Pos=[]  CS0Rot=[]  CS1Pos=[0 0 0]  CS1Rot=[0 0 0]  CS2Pos=[D12_T*ThPos 0 0]  CS2Rot=[0 0 0]  CS3Pos=[0 0 0]  CS3Rot=[0 0 0]  CS4Pos=[]  CS4Rot=[]  CS5Pos=[]  CS5Rot=[]  CS6Pos=[]  CS6Rot=[]  CS7Pos=[]  CS7Rot=[]  CS8Pos=[]  CS8Rot=[]  CS9Pos=[]  CS9Rot=[]  CS10Pos=[]  CS10Rot=[]  CS11Pos=[]  CS11Rot=[]  CS12Pos=[]  CS12Rot=[]  CS13Pos=[]  CS13Rot=[]  CS14Pos=[]  CS14Rot=[]  CS15Pos=[]  CS15Rot=[]  CS16Pos=[]  CS16Rot=[]  CS17Pos=[]  CS17Rot=[]  CS18Pos=[]  CS18Rot=[]  CS19Pos=[]  CS19Rot=[]  CS20Pos=[]  CS20Rot=[]
      settings: SourceProductName=Simscape Multibody  SourceProductBaseCode=MS
  Scope : Scope  Commented=on
  Scope1 : Scope  Commented=on
  Scope5 : Scope
  Selector{3..4,8..9,11..14} (8 alike) : Selector  InputPortWidth=3  IndexOptions=Index vector (dialog)  Indices=[1 3]  OutputSizes=1
  Sum : Sum  Commented=on  Inputs=|++
  Torque : Goto  Commented=on  GotoTag=prosthesis_t  TagVisibility=global
  Unit Delay : UnitDelay  Commented=on  SampleTime=1/Fs_prosthesis
  body pitch/roll/yaw in body frame --- x-axis: forward y-axis: leftward z-axis: parallel to gravity : Subsystem
  "lateral d, v in body frame (left)" : Subsystem
  "lateral d, v in body frame (right)" : Subsystem
  map (-pi,pi] to [0,2pi){,3..7} (6 alike) : Fcn  Expr=u*(u>=0) + (2*pi+u)*(u<0)
  passive ankle : Fcn  Expr=ankleIMP(1)*82*(-u(1)+0.5*pi-ankleIMP(3))-ankleIMP(2)*u(2)
  "sagittal d, v in body frame (left)" : Subsystem
  "sagittal d, v in body frame (right)" : Subsystem
  tag scope: AV_Shank=global, AVl_Shank=global, LKneeState=global, LLBallCnt=global, LLHeelCnt=global, LLLoad=global, LMBallCnt=global, LMHeelCnt=global, L_jrf=global, Lphi12dphi12=global, Lphi23dphi23=global, Lphi34dphi34=global, Lphi34dphi34R=global, RKneeState=global, RLBallCnt=global, RLHeelCnt=global, RLLoad=global, RMBallCnt=global, RMHeelCnt=global, Rphi12dphi12=global, Rphi23dphi23=global, Rphi34dphi34=global, Rphi34dphi34R=global, acc_Shank=global, accl_Shank=global, dtheta=global, dthetaR=global, dxyzHAT=global, dxyzLFoot=global, dxyzLHip=global, dxyzLShank=global, dxyzLThighHigh=global, dxyzLThighLow=global, dxyzRFoot=global, dxyzRHip=global, dxyzRShank=global, dxyzRThighHigh=global, dxyzRThighLow=global, front_dv_L=global, front_dv_R=global, knee_data=global, rotThigh=global, rotTrunk=global, side_dv_L=global, side_dv_R=global, theta=global, thetaR=global, thetaY=global, xyzHAT=global, xyzLAnkle=global, xyzLFoot=global, xyzLHip=global, xyzLKnee=global, xyzLLBall=global, xyzLLHeel=global, xyzLMBall=global, xyzLMHeel=global, xyzLShank=global, xyzLThighHigh=global, xyzLThighLow=global, xyzRAnkle=global, xyzRFoot=global, xyzRHip=global, xyzRKnee=global, xyzRLBall=global, xyzRLHeel=global, xyzRMBall=global, xyzRMHeel=global, xyzRShank=global, xyzRThighHigh=global, xyzRThighLow=global, xyzTrunk=global
  wires:
  [xyzLAnkle] -> Selector9/1
  [xyzRAnkle] -> Selector11/1
  [dxyzHAT] -> Selector4/1
  Selector11/1 -> "lateral d, v in body frame (left)"/2(d0)
  Selector3/1 -> "lateral d, v in body frame (left)"/3(dist), "lateral d, v in body frame (right)"/3(dist)
  Selector4/1 -> "lateral d, v in body frame (left)"/4(vel), "lateral d, v in body frame (right)"/4(vel)
  [thetaY] -> "lateral d, v in body frame (left)"/1(body yaw), "lateral d, v in body frame (right)"/1(body yaw)
  [xyzHAT] -> Selector3/1
  Selector9/1 -> "lateral d, v in body frame (right)"/2(d0)
  body pitch/roll/yaw in body frame --- x-axis: forward y-axis: leftward z-axis: parallel to gravity/1(th_pitch) -> [theta]
  body pitch/roll/yaw in body frame --- x-axis: forward y-axis: leftward z-axis: parallel to gravity/2(dth_pitch) -> [dtheta]
  [xyzLHip] -> body pitch/roll/yaw in body frame --- x-axis: forward y-axis: leftward z-axis: parallel to gravity/1(LHip)
  [dxyzLHip] -> body pitch/roll/yaw in body frame --- x-axis: forward y-axis: leftward z-axis: parallel to gravity/2(dLHip)
  [xyzRHip] -> body pitch/roll/yaw in body frame --- x-axis: forward y-axis: leftward z-axis: parallel to gravity/5(RHip)
  [dxyzRHip] -> body pitch/roll/yaw in body frame --- x-axis: forward y-axis: leftward z-axis: parallel to gravity/6(dRHip)
  [xyzHAT] -> body pitch/roll/yaw in body frame --- x-axis: forward y-axis: leftward z-axis: parallel to gravity/3(HAT)
  [dxyzHAT] -> body pitch/roll/yaw in body frame --- x-axis: forward y-axis: leftward z-axis: parallel to gravity/4(dHAT)
  body pitch/roll/yaw in body frame --- x-axis: forward y-axis: leftward z-axis: parallel to gravity/3(th_roll) -> [thetaR]
  body pitch/roll/yaw in body frame --- x-axis: forward y-axis: leftward z-axis: parallel to gravity/4(dth_roll) -> [dthetaR]
  body pitch/roll/yaw in body frame --- x-axis: forward y-axis: leftward z-axis: parallel to gravity/5(yaw) -> [thetaY]
  "lateral d, v in body frame (left)"/1("d, v") -> L GLU Golgi Tendon Organs5/1
  [xyzLAnkle] -> Selector13/1
  [xyzRAnkle] -> Selector14/1
  [dxyzHAT] -> Selector12/1
  Selector14/1 -> "sagittal d, v in body frame (left)"/2(d0)
  Selector8/1 -> "sagittal d, v in body frame (left)"/3(dist), "sagittal d, v in body frame (right)"/3(dist)
  Selector12/1 -> "sagittal d, v in body frame (left)"/4(vel), "sagittal d, v in body frame (right)"/4(vel)
  [thetaY] -> "sagittal d, v in body frame (left)"/1(body yaw), "sagittal d, v in body frame (right)"/1(body yaw)
  [xyzHAT] -> Selector8/1
  Selector13/1 -> "sagittal d, v in body frame (right)"/2(d0)
  "sagittal d, v in body frame (left)"/1("d, v") -> [front_dv_L]
  "sagittal d, v in body frame (right)"/1("d, v") -> [front_dv_R]
  L GLU Golgi Tendon Organs5/1 -> [side_dv_L]
  "lateral d, v in body frame (right)"/1("d, v") -> [side_dv_R]
  Right Heel Sensor9/1 -> [xyzLHip]
  Right Heel Sensor9/2 -> [dxyzLHip]
  Right Heel Sensor8/2 -> [dxyzRHip]
  Right Heel Sensor8/1 -> [xyzRHip]
  LLHeelCnt4/1(RBallCnt) -> L Heel Skin Load Sensor/1
  L Heel Skin Load Sensor/1 -> [LLHeelCnt]
  L Ball Skin Load Sensor/1 -> [LLBallCnt]
  LLHeelCnt2/1(RBallCnt) -> L Ball Skin Load Sensor/1
  Left Thigh Sensor Sheet/1(dx) -> L Thigh Displacement  Sensor/1
  L Thigh Displacement  Sensor/1 -> Left Leg Load/1(dxThigh [m])
  map (-pi,pi] to [0,2pi)6/1 -> Mux4/1
  LeftKnee Sensor/2 -> Mux4/2
  LeftKnee Sensor/1 -> map (-pi,pi] to [0,2pi)6/1
  Mux4/1 -> [Lphi23dphi23], L Knee Joint Sensor/1
  map (-pi,pi] to [0,2pi)3/1 -> Mux6/1
  Left Ankle Sensor/2 -> Mux6/2
  Left Ankle Sensor/1 -> map (-pi,pi] to [0,2pi)3/1
  Mux6/1 -> passive ankle/1, [Lphi12dphi12]
  L Knee Joint Sensor/1 -> [LKneeState]
  [RM12] -> Right Ankle Actuator/1
  Right Thigh Sensor Sheet/1(dx) -> R Thigh Displacement  Sensor/1
  R Thigh Displacement  Sensor/1 -> Right Leg Load/1(dxThigh [m])
  map (-pi,pi] to [0,2pi)4/1 -> Mux5/1
  Right Knee Sensor/2 -> Mux5/2
  Mux5/1 -> [Rphi23dphi23], R Knee Joint Sensor/1
  Right Knee Sensor/1 -> map (-pi,pi] to [0,2pi)4/1
  map (-pi,pi] to [0,2pi)7/1 -> Mux7/1
  Right Ankle Sensor/2 -> Mux7/2
  Right Ankle Sensor/1 -> map (-pi,pi] to [0,2pi)7/1
  Mux7/1 -> [Rphi12dphi12]
  R Knee Joint Sensor/1 -> [RKneeState]
  Right Heel Sensor14/1 -> [xyzRKnee]
  RAnkle/1(Pos) -> [xyzRAnkle]
  map (-pi,pi] to [0,2pi)/1 -> Mux2/1
  Left Hip Sensor/2 -> Mux2/2
  Left Hip Sensor/1 -> map (-pi,pi] to [0,2pi)/1
  Mux2/1 -> [Lphi34dphi34]
  Left Hip Sensor (roll)/2 -> Mux14/2
  Left Hip Sensor (roll)/1 -> Mux14/1
  Mux14/1 -> [Lphi34dphi34R]
  [LM34R] -> Left Hip Actuator (roll)/1
  map (-pi,pi] to [0,2pi)5/1 -> Mux3/1
  Right Hip Sensor/2 -> Mux3/2
  Right Hip Sensor/1 -> map (-pi,pi] to [0,2pi)5/1
  Mux3/1 -> [Rphi34dphi34]
  Right Hip Sensor (roll)/2 -> Mux15/2
  Right Hip Sensor (roll)/1 -> Mux15/1
  Mux15/1 -> L GLU Golgi Tendon Organs3/1
  [RM34R] -> L GLU Golgi Tendon Organs1/1
  L GLU Golgi Tendon Organs3/1 -> [Rphi34dphi34R]
  L GLU Golgi Tendon Organs1/1 -> Right Hip Actuator (roll)/1
  Right Heel Sensor21/1 -> [xyzLLBall]
  Right Heel Sensor20/1 -> [xyzLMBall]
  Right Heel Sensor23/1 -> [xyzLLHeel]
  Right Heel Sensor12/1 -> [xyzRLHeel]
  Right Heel Sensor10/1 -> [xyzRMHeel]
  Right Heel Sensor3/1 -> [xyzRLBall]
  Right Heel Sensor13/1 -> [xyzRMBall]
  LLHeelCnt1/1(RBallCnt) -> L Heel Skin Load Sensor1/1
  L Heel Skin Load Sensor1/1 -> [LMHeelCnt]
  L Ball Skin Load Sensor1/1 -> [LMBallCnt]
  LLHeelCnt3/1(RBallCnt) -> L Ball Skin Load Sensor1/1
  LLHeelCnt8/1(RBallCnt) -> L Heel Skin Load Sensor2/1
  LLHeelCnt5/1(RBallCnt) -> L Heel Skin Load Sensor3/1
  LLHeelCnt7/1(RBallCnt) -> L Ball Skin Load Sensor3/1
  LLHeelCnt6/1(RBallCnt) -> L Ball Skin Load Sensor2/1
  L Heel Skin Load Sensor2/1 -> [RLHeelCnt]
  L Heel Skin Load Sensor3/1 -> [RMHeelCnt]
  L Ball Skin Load Sensor3/1 -> [RMBallCnt]
  L Ball Skin Load Sensor2/1 -> [RLBallCnt]
  Right Heel Sensor6/1 -> [xyzLKnee]
  Right Leg Load/1(LLoad [F]) -> [RLLoad]
  Add/1 -> Left Knee Actuator/1
  [LM23_D] -> Add/2
  [LM34_D] -> Add1/2
  Add1/1 -> Left Hip Actuator/1
  [LM34] -> Add1/1
  [RM34_D] -> Add2/2
  Add2/1 -> Right Hip Actuator/1
  [RM34] -> Add2/1
  [RM23] -> Add3/1
  Add3/1 -> Right Knee Actuator/1
  [RM23_D] -> Add3/2
  [xyzHAT_D_sag] -> RLBall Cnt1/1(Dist_sag)
  [xyzRAnkle_D] -> RAnkle/1(Dist)
  LAnkle/1(Pos) -> [xyzLAnkle]
  [xyzLAnkle_D] -> LAnkle/1(Dist)
  [xyzHAT_D_front] -> RLBall Cnt1/2(Dist_front)
  Right Heel Sensor5/1 -> [xyzHAT]
  Right Heel Sensor5/2 -> [dxyzHAT]
  RLBall Cnt1/1(Pos) -> [xyzTrunk]
  RLBall Cnt1/2(Rot) -> [rotTrunk]
  Right Heel Sensor1/1 -> [xyzLThighHigh]
  Right Heel Sensor2/1 -> [xyzLThighLow]
  Right Heel Sensor4/1 -> [xyzLShank]
  Right Heel Sensor7/1 -> [xyzLFoot]
  Right Heel Sensor15/1 -> [xyzRThighLow]
  Right Heel Sensor11/1 -> [xyzRThighHigh]
  Right Heel Sensor16/1 -> [xyzRShank]
  Right Heel Sensor17/1 -> [xyzRFoot]
  Right Heel Sensor11/2 -> [dxyzRThighHigh]
  Right Heel Sensor15/2 -> [dxyzRThighLow]
  Right Heel Sensor16/2 -> [dxyzRShank]
  Right Heel Sensor17/2 -> [dxyzRFoot]
  Right Heel Sensor7/2 -> [dxyzLFoot]
  Right Heel Sensor4/2 -> [dxyzLShank]
  Right Heel Sensor1/2 -> [dxyzLThighHigh]
  Right Heel Sensor2/2 -> [dxyzLThighLow]
  Left Leg Load/1(LLoad [F]) -> [LLLoad]
  Right Heel Sensor22/1 -> [xyzLMHeel]
  LLHeelCnt4/2(RBallCnt1) -> LLHeelCnt1/1(PosContra)
  LLHeelCnt3/2(RBallCnt1) -> LLHeelCnt2/1(PosContra)
  LLHeelCnt8/2(RBallCnt1) -> LLHeelCnt5/1(PosContra)
  LLHeelCnt7/2(RBallCnt1) -> LLHeelCnt6/1(PosContra)
  LeftKnee Sensor/3 -> [L_jrf]
  [acc_Shank] -> Matrix Concatenate/1
  [AV_Shank] -> Matrix Concatenate/2
  [Lphi23dphi23] -> Matrix Concatenate/3
  [L_jrf] -> Matrix Concatenate/4
  [LLBallF] -> Matrix Concatenate/5
  [LMBallF] -> Matrix Concatenate/6
  [LLHeelF] -> Matrix Concatenate/7
  [LMHeelF] -> Matrix Concatenate/8
  Matrix Concatenate/1 -> [knee_data]
  Left Knee Moment13/1 -> MATLAB Function1/1(u)
  MATLAB Function1/1(y) -> MATLAB Function/1(signal), HAT Position34/1
  [LM23] -> Add/1
  Unit Delay/1 -> Torque/1
  Left Knee Moment11/1 -> MATLAB Function/2(tNMC)
  MATLAB Function/3(t_stop) -> Sum/2
  Sum/1 -> Unit Delay/1
  MATLAB Function/1(t) -> Scope1/1, Sum/1
  [LM12] -> Manual Switch1/2
  Manual Switch1/1 -> Left Ankle Actuator/1
  passive ankle/1 -> Manual Switch1/1
  MATLAB Function/2(state) -> Scope/1
  Constant/1 -> MATLAB Function/3(type)
  Right Heel Sensor4/4 -> [acc_Shank]
  Right Heel Sensor4/3 -> [AV_Shank], Scope5/1
  [accl_Shank] -> Matrix Concatenate/9
  [AVl_Shank] -> Matrix Concatenate/10
  Right Heel Sensor18/1 -> [AVl_Shank]
  Right Heel Sensor18/2 -> [accl_Shank]
  Right Heel Sensor2/3 -> [rotThigh]
  [rotThigh] -> Matrix Concatenate/11
  connections:
  HAT/RConn4 -- Right Hip Joint1/RConn1
  Left Hip Joint1/RConn2 -- Left Hip IC/RConn1
  Left Thigh High/RConn1 -- Left Thigh Sensor Sheet/RConn1
  LLHeelCnt5/LConn1 -- Right Foot/RConn5
  RLBall Cnt1/LConn1 -- HAT/LConn2
  Right Knee Actuator/RConn1 -- Right Knee Joint/LConn2
  HAT/RConn1 -- Left Hip Joint1/RConn1
  Right Thigh Sensor Sheet/RConn1 -- Right Thigh Low/RConn1
  Right Thigh Sensor Sheet/LConn1 -- Right Thigh High/LConn2
  Right Knee Joint/RConn2 -- Right Knee IC/RConn1
  6 DOF/LConn1 -- Ground/RConn1
  LLHeelCnt4/LConn1 -- Left Foot/RConn5
  Left Knee Joint/RConn1 -- Left Thigh Low/RConn2
  Right Foot/RConn2 -- Right Heel Sensor12/LConn1
  Right Foot/RConn3 -- Right Ankle Joint/LConn1
  LLHeelCnt1/LConn1 -- Left Foot/RConn6
  Right Ankle Joint/RConn1 -- Right Shank/LConn2
  Left Foot/RConn2 -- Right Heel Sensor22/LConn1
  Left Foot/RConn4 -- Left Ankle Joint/LConn1
  Left Knee Joint/LConn2 -- Left Knee Actuator/RConn1
  Right Knee Joint/LConn3 -- Right Knee Sensor/LConn1
  Left Foot/LConn2 -- Right Heel Sensor21/LConn1
  Left Knee Joint/RConn2 -- Left Knee IC/RConn1
  Right Hip IC/RConn1 -- Right Hip Joint1/RConn2
  Left Hip Sensor (roll)/LConn1 -- Left Hip Joint1/RConn3
  Left Hip Joint1/LConn3 -- Left Hip Sensor/LConn1
  Right Hip Joint1/LConn3 -- Right Hip Sensor/LConn1
  HAT/RConn3 -- Right Heel Sensor8/LConn1
  Left Ankle Joint/LConn2 -- Left Ankle Actuator/RConn1
  Left Hip Joint1/LConn1 -- Left Thigh High/LConn2
  6 DOF/LConn2 -- Left Ball IC/RConn1
  Left Ankle Sensor/LConn1 -- Left Ankle Joint/LConn3
  Right Foot/LConn3 -- Right Heel Sensor3/LConn1
  LLHeelCnt7/LConn1 -- Right Foot/LConn6
  LLHeelCnt3/LConn1 -- Left Foot/LConn5
  Right Shank/RConn2 -- Right Knee Joint/LConn1
  Left Ankle Joint/RConn2 -- Left Ankle IC/RConn1
  Right Hip Joint1/LConn1 -- Right Thigh High/RConn1
  LeftKnee Sensor/LConn1 -- Left Knee Joint/LConn3
  Right Hip Joint1/LConn2 -- Right Hip Actuator/RConn1
  Left Shank/RConn2 -- Left Knee Joint/LConn1
  HAT/RConn2 -- Right Heel Sensor9/LConn1
  Right Hip Actuator (roll)/RConn1 -- Right Hip Joint1/LConn4
  Right Ankle Joint/LConn3 -- Right Ankle Sensor/LConn1
  Right Ankle Joint/RConn2 -- Right Ankle IC/RConn1
  LLHeelCnt6/LConn1 -- Right Foot/LConn5
  Ground/LConn1 -- Machine Environment/RConn1
  Left Thigh Sensor Sheet/LConn1 -- Left Thigh Low/LConn2
  Left Thigh Low/RConn1 -- Right Heel Sensor6/LConn1
  Right Ankle Actuator/RConn1 -- Right Ankle Joint/LConn2
  Left Hip Actuator (roll)/RConn1 -- Left Hip Joint1/LConn4
  Right Thigh Low/LConn2 -- Right Heel Sensor14/LConn1
  Left Foot/RConn3 -- Right Heel Sensor23/LConn1
  Left Hip Joint1/LConn2 -- Left Hip Actuator/RConn1
  Left Foot/LConn3 -- 6 DOF/RConn1
  RAnkle/LConn1 -- Right Shank/LConn1
  Right Hip Sensor (roll)/LConn1 -- Right Hip Joint1/RConn3
  Left Ankle Joint/RConn1 -- Left Shank/LConn3
  Right Knee Joint/RConn1 -- Right Thigh Low/LConn3
  LLHeelCnt8/LConn1 -- Right Foot/RConn4
  Right Foot/LConn2 -- Right Heel Sensor13/LConn1
  Left Foot/LConn1 -- Right Heel Sensor20/LConn1
  Right Heel Sensor10/LConn1 -- Right Foot/RConn1
  Left Shank/LConn2 -- LAnkle/LConn1
  HAT/LConn1 -- Right Heel Sensor5/LConn1
  Right Heel Sensor1/LConn1 -- Left Thigh High/LConn1
  Right Heel Sensor2/LConn1 -- Left Thigh Low/LConn1
  Right Heel Sensor7/LConn1 -- Left Foot/RConn1
  Right Heel Sensor15/LConn1 -- Right Thigh Low/LConn1
  Right Heel Sensor11/LConn1 -- Right Thigh High/LConn1
  Right Heel Sensor16/LConn1 -- Right Shank/RConn1
  Right Heel Sensor17/LConn1 -- Right Foot/LConn1
  Left Shank/LConn1 -- Right Heel Sensor4/LConn1
  LLHeelCnt2/LConn1 -- Left Foot/LConn4
  Left Shank/RConn1 -- Right Heel Sensor18/LConn1
